simulink model "topic1msd"  (R2024b)
settings: Solver=VariableStepAuto  StartTime=0.0  StopTime=10.0  RelTol=1e-3
values from neighbouring files (symbols this model uses):
  c = 1    [workshop1.m]
  k = 10    [workshop1.m]
  m = 2    [workshop1.m]
settings Model: Creator=will  LastModifiedBy=will

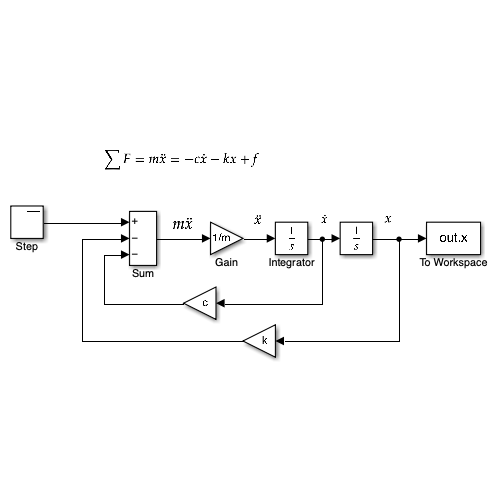
[thumbnail: Simulink's stored preview of the top-level diagram]
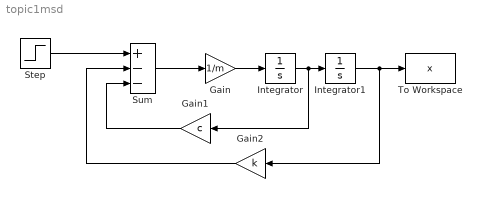
== system topic1msd ==
  Gain : Gain  Gain=1/m
  Gain1 : Gain  Gain=c
  Gain2 : Gain  Gain=k
  Integrator : Integrator
  Integrator1 : Integrator
  Step : Step  SampleTime=0
  Sum : Sum  Inputs=+--
  To Workspace : ToWorkspace  VariableName=x  SaveFormat=Timeseries  SampleTime=-1
  wires:
  Step/1 -> Sum/1
  Sum/1 -> Gain/1
  Gain/1 -> Integrator/1
  Integrator/1 -> Integrator1/1, Gain1/1
  Integrator1/1 -> To Workspace/1, Gain2/1
  Gain1/1 -> Sum/3
  Gain2/1 -> Sum/2
